simulink model "MotorTest"  (R2015a)
settings: Solver=ode3  StartTime=0.0  StopTime=10.0  FixedStep=1/200  RelTol=1e-3
undefined symbols (not defined in the file): Ch, gamma, Kh, L, M1, R
libraries: PoliArd x6
settings Model: ExtModeTrigDuration=2  Creator=User  LastModifiedBy=user
settings OptimizationCC: OptimizeModelRefInitCode=on  LifeSpan=1
settings DebuggingCC: UnderspecifiedInitializationDetection=Classic  MergeDetectMultiDrivingBlocksExec=none
settings HardwareCC: ProdLargestAtomicInteger=Long  ProdLargestAtomicFloat=Double  ProdEndianess=LittleEndian  ProdHWDeviceType=ARM Compatible->ARM Cortex
settings RTWCC: SystemTargetFile=realtime.tlc  GenerateMakefile=off  TemplateMakefile=realtime.tmf  Description=Run on Target Hardware  RTWVerbose=off
settings ERTTargetCC: CombineOutputUpdateFcns=off  ExtModeTransport=3  ExtModeMexFile=ext_serial_win32_comm_rtt  ExtModeMexArgs=0 1 9600  ERTSrcFileBannerTemplate=realtime_code_template.cgt  ERTHdrFileBannerTemplate=realtime_code_template.cgt  ERTDataSrcFileTemplate=realtime_code_template.cgt  ERTDataHdrFileTemplate=realtime_code_template.cgt  ERTCustomFileTemplate=realtime_file_process.tlc

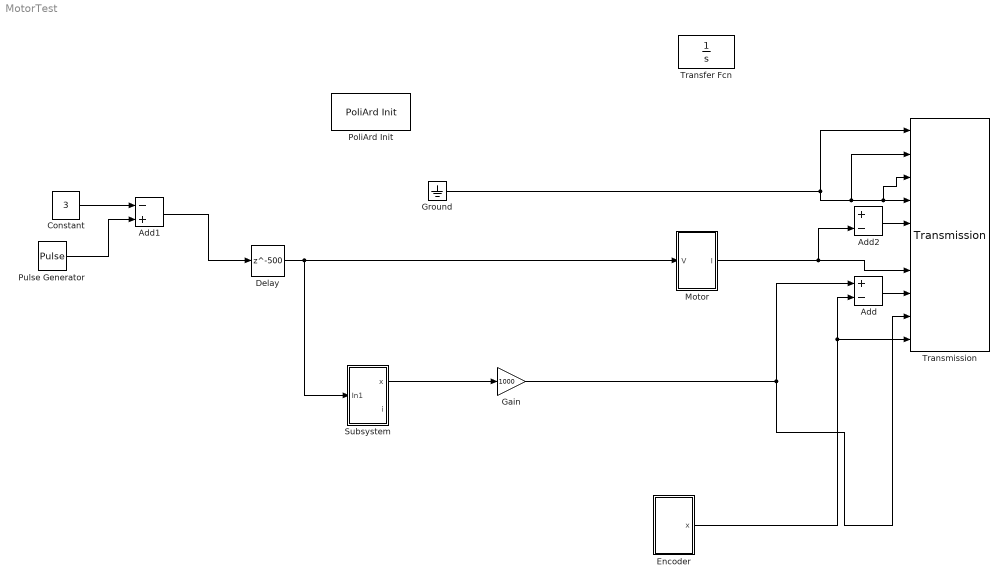
== system MotorTest ==
  Add : Sum  Inputs=+-
  Add1 : Sum  Inputs=-+
  Add2 : Sum  Inputs=+-
  Constant : Constant  Value=3
  Delay : Delay  DelayLength=500
  "Encoder " : Subsystem
  Gain : Gain  Gain=1000
  Ground : Ground
  Motor : Subsystem
  PoliArd Init : PoliArd/PoliArd Init
  Pulse Generator : DiscretePulseGenerator  PulseType=Time based  Amplitude=6  Period=10  PulseWidth=50  PhaseDelay=5
  Subsystem : Subsystem
  Transfer Fcn : TransferFcn  Denominator=[1 0]
  Transmission : PoliArd/Transmission  sample_freq=200  sig_to_send=6
  wires:
  Ground/1 -> Transmission/2, Transmission/3, Transmission/4, Transmission/1
  Motor/1(I) -> Add2/2, Transmission/7
  "Encoder "/1(x) -> Add/2, Transmission/10
  Add/1 -> Transmission/8
  Constant/1 -> Add1/1
  Pulse Generator/1 -> Add1/2
  Add2/1 -> Transmission/5
  Delay/1 -> Subsystem/1(In1), Motor/1(V)
  Add1/1 -> Delay/1
  Subsystem/1(x) -> Gain/1
  Gain/1 -> Add/1, Transmission/9

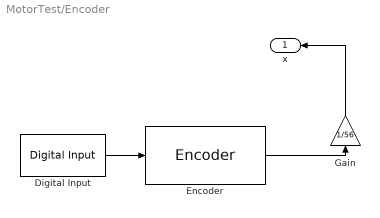
== system MotorTest/Encoder  ==
  Digital Input : PoliArd/Digital Input  DI_pin=2  DIsample=1/200
  Encoder : PoliArd/Encoder  EncoderID=1  dt_enc=-1
  Gain : Gain  Gain=1/56
  x : Outport
  wires:
  Digital Input/1 -> Encoder/1
  Encoder/1 -> Gain/1
  Gain/1 -> x/1

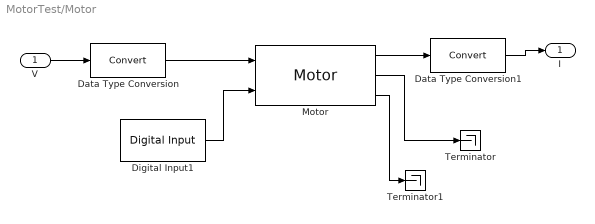
== system MotorTest/Motor ==
  V : Inport
  Data Type Conversion : DataTypeConversion
  Data Type Conversion1 : DataTypeConversion
  Digital Input1 : PoliArd/Digital Input  DI_pin=3  DIsample=1/200
  Motor : PoliArd/Motor  MotorID=1  DC_bus_mask=12  dt_mot=1/200
  Terminator : Terminator
  Terminator1 : Terminator
  I : Outport
  wires:
  Data Type Conversion/1 -> Motor/1
  Digital Input1/1 -> Motor/2
  V/1 -> Data Type Conversion/1
  Motor/3 -> Terminator1/1
  Motor/2 -> Terminator/1
  Motor/1 -> Data Type Conversion1/1
  Data Type Conversion1/1 -> I/1

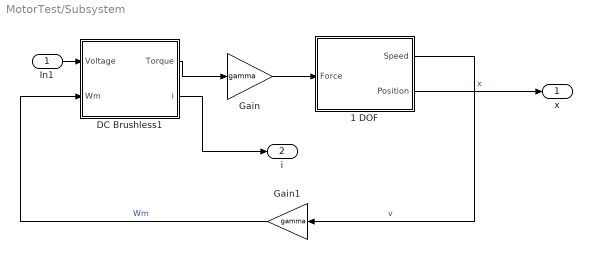
== system MotorTest/Subsystem ==
  In1 : Inport
  "1 DOF " : Subsystem
  DC Brushless1 : Subsystem
  Gain : Gain  Gain=gamma
  Gain1 : Gain  Gain=gamma
  x : Outport
  "i " : Outport  Port=2
  wires:
  "1 DOF "/2("Position ") -> x/1  "x"
  Gain/1 -> "1 DOF "/1(Force)
  "1 DOF "/1("Speed ") -> Gain1/1  "v"
  Gain1/1 -> DC Brushless1/2(Wm)  "Wm"
  DC Brushless1/1("Torque ") -> Gain/1
  DC Brushless1/2("i ") -> "i "/1
  In1/1 -> DC Brushless1/1("Voltage ")

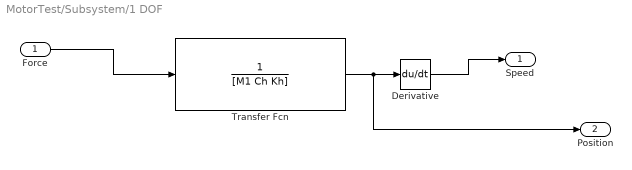
== system MotorTest/Subsystem/1 DOF  ==
  Force : Inport
  Derivative : Derivative
  Transfer Fcn : TransferFcn  Denominator=[M1 Ch Kh]
  "Speed " : Outport
  "Position " : Outport  Port=2
  wires:
  Force/1 -> Transfer Fcn/1
  Transfer Fcn/1 -> "Position "/1, Derivative/1
  Derivative/1 -> "Speed "/1

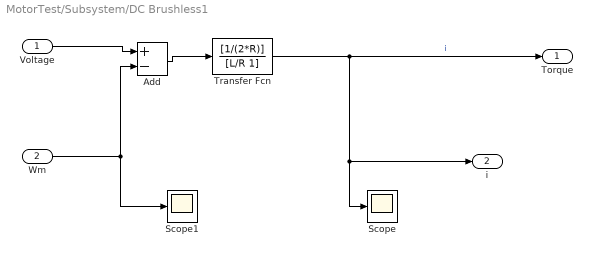
== system MotorTest/Subsystem/DC Brushless1 ==
  "Voltage " : Inport
  Wm : Inport  Port=2
  Add : Sum  Inputs=+-
  Scope : Scope
      settings: YMin=-0.075  YMax=0.125  SaveName=ScopeData2
  Scope1 : Scope
      settings: YMin=-0.35  YMax=0.35  SaveName=ScopeData4
  Transfer Fcn : TransferFcn  Numerator=[1/(2*R)]  Denominator=[L/R 1]
  "Torque " : Outport
  "i " : Outport  Port=2
  wires:
  Transfer Fcn/1 -> "Torque "/1, "i "/1, Scope/1  "i"
  Add/1 -> Transfer Fcn/1
  "Voltage "/1 -> Add/1
  Wm/1 -> Scope1/1, Add/2
